simulink model "RC_plant_PI_controller_simulation"  (R2024b)
settings: Solver=ode4  StartTime=0.0  StopTime=10.0  FixedStep=0.001  RelTol=1e-3
libraries: cstblocks x2
settings Model: Creator=User  LastModifiedBy=User

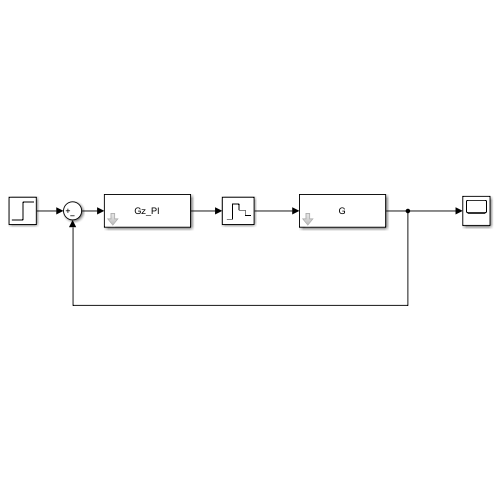
[thumbnail: Simulink's stored preview of the top-level diagram]
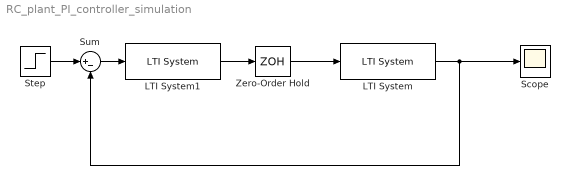
== system RC_plant_PI_controller_simulation ==
  LTI System : cstblocks/LTI System  sys=G  IC=[]  PadeOrder=0
  LTI System1 : cstblocks/LTI System  sys=Gz_PI  IC=[]  PadeOrder=0
  Scope : Scope
  Step : Step  Time=0  SampleTime=0
  Sum : Sum  Inputs=|+-
  Zero-Order Hold : ZeroOrderHold  SampleTime=-1
  wires:
  Sum/1 -> LTI System1/1
  LTI System/1 -> Scope/1, Sum/2
  Step/1 -> Sum/1
  Zero-Order Hold/1 -> LTI System/1
  LTI System1/1 -> Zero-Order Hold/1
